simulink library "halout"  (R2021b)
settings: Solver=VariableStepAuto  StartTime=0.0  StopTime=10.0  RelTol=1e-3
undefined symbols (not defined in the file): C_TASK_5MS_S, FALSE, KHAL_CAN1FD1APS3E2E_flg, KHAL_CAN1FD1APS3TxReq_flg, KHAL_CAN1FD1VCU2E2E_flg, KHAL_CAN1FD1VCU2TxReq_flg, KHAL_CAN1FD1VCU3E2E_flg, KHAL_CAN1FD1VCU3TxReq_flg, KHAL_CAN1TxReq_flg, KHAL_CAN1VMCFCM1E2E_flg, KHAL_CAN1VMCFCM1TxReq_flg, KHAL_CAN2TxReq_flg, KHAL_CAN3FD3VCU1toNIDECTxReq_flg, KHAL_CAN3FD3VCU1TxReq_flg, KHAL_CAN3FD3VCU2E2E_flg, KHAL_CAN3FD3VCU2toNIDECE2E_flg, KHAL_CAN3FD3VCU2toNIDECTxReq_flg, KHAL_CAN3FD3VCU2TxReq_flg, KHAL_CAN3TxReq_flg, KHAL_CAN4FD4CE1000E2E_flg, KHAL_CAN4FD4CE1000TxReq_flg, KHAL_CAN4TxReq_flg, KHAL_CAN5TxReq_flg, KHAL_CAN6FD6APS3E2E_flg, KHAL_CAN6FD6APS3TxReq_flg, KHAL_CAN6FD6VCU2E2E_flg, KHAL_CAN6FD6VCU2TxReq_flg, KHAL_CAN6TxReq_flg, ONE_INT, TRUE, ZERO_INT
libraries: FVT_lib x549, simulink x244
(part 9 of 27)

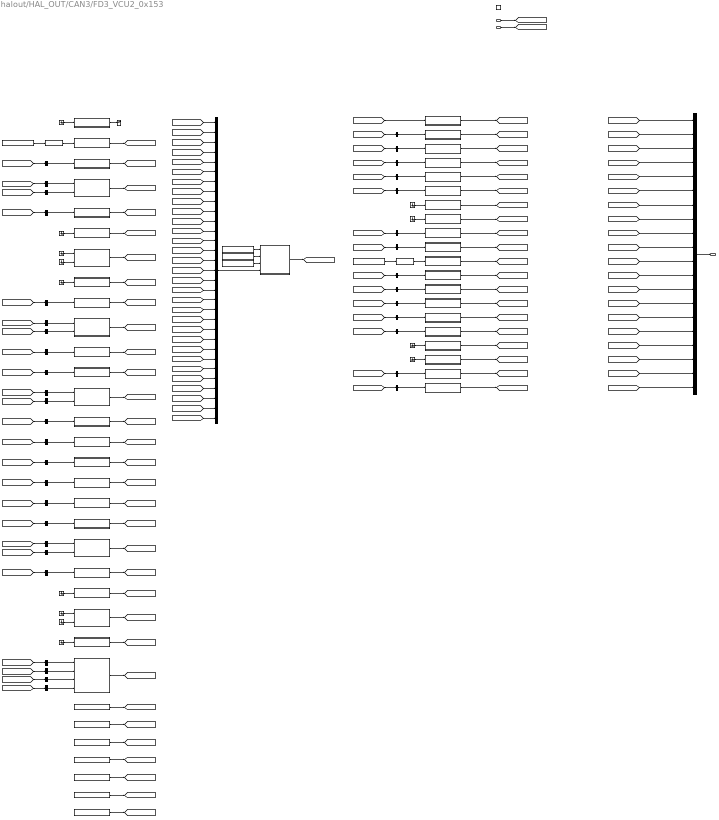
== system halout/HAL_OUT/CAN3/FD3_VCU2_0x153 ==
  BSCP_outputs : Inport  OutDataTypeStr=Bus: BSCP_outputs
  BOUTP_outputs : Inport  Port=2  OutDataTypeStr=Bus: BOUTP_outputs
  Trigger : TriggerPort  TriggerType=function-call  VariantControl=(inherit)
  Byte_0 : Subsystem
  Byte_1 : Subsystem
  Byte_10 : Subsystem
  Byte_11 : Subsystem
  Byte_12 : Subsystem
  Byte_13 : Subsystem
  Byte_14 : Subsystem
  Byte_15 : Subsystem
  Byte_16 : Subsystem
  Byte_17 : Subsystem
  Byte_18 : Subsystem
  Byte_19 : Subsystem
  Byte_2 : Subsystem
  Byte_20 : Subsystem
  Byte_21 : Subsystem
  Byte_22 : Subsystem
  Byte_23 : Subsystem
  Byte_24 : Subsystem
  Byte_{25..31} (7 alike) : Constant  Value=ZERO_INT
  Byte_3 : Subsystem
  Byte_4 : Subsystem
  Byte_5 : Subsystem
  Byte_6 : Subsystem
  Byte_7 : Subsystem
  Byte_8 : Subsystem
  Byte_9 : Subsystem
  CRC8_IfAction_Tx : Subsystem  AncestorBlock=FVT_lib/hal/CRC8_IfAction_Tx
      mask help: MeasumentTrigerEvent
      mask Display: fprintf('CRC8_IfAction');
  CSVCU2CAN1 : Subsystem
  Constant : Constant  Value=KHAL_CAN3FD3VCU2E2E_flg
  Constant1 : Constant  Value=0x40
  Constant2 : Constant  Value=0x24
  Constant3 : Constant  Value=KHAL_CAN3FD3VCU2E2E_flg
  Constant4 : Constant  Value=KHAL_CAN3FD3VCU2E2E_flg
  FrActvDmpDisabReq : Subsystem
  FrIdcMax : Subsystem
  FrIdcMin : Subsystem
  FrMCUEnaReq : Subsystem
  FrTMTqReq : Subsystem
  FrTorqMax : Subsystem
  FrTorqMin : Subsystem
  FrUdcMax : Subsystem
  FrUdcMin : Subsystem
  Ground{,1..12} (13 alike) : Ground
  Mux2 : Mux  Inputs=31
  RCVCU2CAN1 : Subsystem
  RollingCounter_IfAction : FVT_lib/hal/RollingCounter_IfAction
  RollingCounter_IfAction1 : FVT_lib/hal/RollingCounter_IfAction
  RrActvDmpDisabReq : Subsystem
  RrIdcMax : Subsystem
  RrIdcMin : Subsystem
  RrMCUEnaReq : Subsystem
  RrTMTqReq : Subsystem
  RrTorqMax : Subsystem
  RrTorqMin : Subsystem
  RrUdcMax : Subsystem
  RrUdcMin : Subsystem
  Terminator : Terminator
  bus_creator : BusCreator  Inputs=20  OutDataTypeStr=Bus: DT_CAN3_SG_FD3_VCU2  NonVirtualBus=on
  bus_selector : BusSelector  OutputSignals=VOUTP_RrIdcMax_A
  bus_selector1 : BusSelector  OutputSignals=VOUTP_RrIdcMax_A
  bus_selector10 : BusSelector  OutputSignals=VOUTP_FrUdcMin_V
  bus_selector11 : BusSelector  OutputSignals=VOUTP_FrUdcMin_V
  bus_selector12 : BusSelector  OutputSignals=VOUTP_RrTMTqReq_Nm
  bus_selector13 : BusSelector  OutputSignals=VOUTP_RrTMTqReq_Nm
  bus_selector14 : BusSelector  OutputSignals=VOUTP_FrTMTqReq_Nm
  bus_selector15 : BusSelector  OutputSignals=VOUTP_FrTMTqReq_Nm
  bus_selector16 : BusSelector  OutputSignals=VOUTP_FrIdcMax_A
  bus_selector17 : BusSelector  OutputSignals=VOUTP_FrIdcMax_A
  bus_selector18 : BusSelector  OutputSignals=VOUTP_FrIdcMin_A
  bus_selector19 : BusSelector  OutputSignals=VOUTP_FrIdcMin_A
  bus_selector2 : BusSelector  OutputSignals=VOUTP_RrIdcMin_A
  bus_selector20 : BusSelector  OutputSignals=VOUTP_FrActvDmpDisabReq_flg
  bus_selector21 : BusSelector  OutputSignals=VOUTP_FrMCUEnaReq_flg
  bus_selector22 : BusSelector  OutputSignals=VOUTP_RrActvDmpDisabReq_flg
  bus_selector23 : BusSelector  OutputSignals=VOUTP_RrMCUEnaReq_flg
  bus_selector24 : BusSelector  OutputSignals=VOUTP_FrActvDmpDisabReq_flg
  bus_selector25 : BusSelector  OutputSignals=VOUTP_FrIdcMax_A
  bus_selector26 : BusSelector  OutputSignals=VOUTP_FrIdcMin_A
  bus_selector27 : BusSelector  OutputSignals=VOUTP_FrMCUEnaReq_flg
  bus_selector28 : BusSelector  OutputSignals=VOUTP_FrTMTqReq_Nm
  bus_selector29 : BusSelector  OutputSignals=VOUTP_FrUdcMax_V
  bus_selector3 : BusSelector  OutputSignals=VOUTP_RrIdcMin_A
  bus_selector30 : BusSelector  OutputSignals=VOUTP_FrUdcMin_V
  bus_selector31 : BusSelector  OutputSignals=VOUTP_RrActvDmpDisabReq_flg
  bus_selector32 : BusSelector  OutputSignals=VOUTP_RrIdcMax_A
  bus_selector33 : BusSelector  OutputSignals=VOUTP_RrIdcMin_A
  bus_selector34 : BusSelector  OutputSignals=VOUTP_RrMCUEnaReq_flg
  bus_selector35 : BusSelector  OutputSignals=VOUTP_RrTMTqReq_Nm
  bus_selector36 : BusSelector  OutputSignals=VOUTP_RrUdcMax_V
  bus_selector37 : BusSelector  OutputSignals=VOUTP_RrUdcMin_V
  bus_selector4 : BusSelector  OutputSignals=VOUTP_RrUdcMax_V
  bus_selector5 : BusSelector  OutputSignals=VOUTP_RrUdcMax_V
  bus_selector6 : BusSelector  OutputSignals=VOUTP_RrUdcMin_V
  bus_selector7 : BusSelector  OutputSignals=VOUTP_RrUdcMin_V
  bus_selector8 : BusSelector  OutputSignals=VOUTP_FrUdcMax_V
  bus_selector9 : BusSelector  OutputSignals=VOUTP_FrUdcMax_V
  FD3_VCU2 : Outport
  wires:
  BSCP_outputs/1 -> [BSCP_outputs]
  BOUTP_outputs/1 -> [BOUTP_outputs]
  [CAN3_CS_VCU2_CAN1] -> bus_creator/1  "CAN3_CS_VCU2_CAN1"
  [CAN3_Fr_ActvDmpDisabReq] -> bus_creator/2  "CAN3_Fr_ActvDmpDisabReq"
  [CAN3_Fr_IdcMax] -> bus_creator/3  "CAN3_Fr_IdcMax"
  [CAN3_Fr_IdcMin] -> bus_creator/4  "CAN3_Fr_IdcMin"
  [CAN3_Fr_MCUEnaReq] -> bus_creator/5  "CAN3_Fr_MCUEnaReq"
  [CAN3_Fr_TMTqReq] -> bus_creator/6  "CAN3_Fr_TMTqReq"
  [CAN3_Fr_TorqMax] -> bus_creator/7  "CAN3_Fr_TorqMax"
  [CAN3_Fr_TorqMin] -> bus_creator/8  "CAN3_Fr_TorqMin"
  [CAN3_Fr_UdcMax] -> bus_creator/9  "CAN3_Fr_UdcMax"
  [CAN3_Fr_UdcMin] -> bus_creator/10  "CAN3_Fr_UdcMin"
  [CAN3_RC_VCU2_CAN1] -> bus_creator/11  "CAN3_RC_VCU2_CAN1"
  [CAN3_Rr_ActvDmpDisabReq] -> bus_creator/12  "CAN3_Rr_ActvDmpDisabReq"
  [CAN3_Rr_IdcMax] -> bus_creator/13  "CAN3_Rr_IdcMax"
  [CAN3_Rr_IdcMin] -> bus_creator/14  "CAN3_Rr_IdcMin"
  [CAN3_Rr_MCUEnaReq] -> bus_creator/15  "CAN3_Rr_MCUEnaReq"
  [CAN3_Rr_TMTqReq] -> bus_creator/16  "CAN3_Rr_TMTqReq"
  [CAN3_Rr_TorqMax] -> bus_creator/17  "CAN3_Rr_TorqMax"
  [CAN3_Rr_TorqMin] -> bus_creator/18  "CAN3_Rr_TorqMin"
  [CAN3_Rr_UdcMax] -> bus_creator/19  "CAN3_Rr_UdcMax"
  [CAN3_Rr_UdcMin] -> bus_creator/20  "CAN3_Rr_UdcMin"
  bus_creator/1 -> FD3_VCU2/1
  CSVCU2CAN1/1(CAN3_CS_VCU2_CAN1) -> [CAN3_CS_VCU2_CAN1]
  FrActvDmpDisabReq/1(CAN3_Fr_ActvDmpDisabReq) -> [CAN3_Fr_ActvDmpDisabReq]
  FrIdcMax/1(CAN3_Fr_IdcMax) -> [CAN3_Fr_IdcMax]
  FrIdcMin/1(CAN3_Fr_IdcMin) -> [CAN3_Fr_IdcMin]
  FrMCUEnaReq/1(CAN3_Fr_MCUEnaReq) -> [CAN3_Fr_MCUEnaReq]
  FrTMTqReq/1(CAN3_Fr_TMTqReq) -> [CAN3_Fr_TMTqReq]
  FrTorqMax/1(CAN3_Fr_TorqMax) -> [CAN3_Fr_TorqMax]
  FrTorqMin/1(CAN3_Fr_TorqMin) -> [CAN3_Fr_TorqMin]
  FrUdcMax/1(CAN3_Fr_UdcMax) -> [CAN3_Fr_UdcMax]
  FrUdcMin/1(CAN3_Fr_UdcMin) -> [CAN3_Fr_UdcMin]
  RCVCU2CAN1/1(CAN3_RC_VCU2_CAN1) -> [CAN3_RC_VCU2_CAN1]
  RrActvDmpDisabReq/1(CAN3_Rr_ActvDmpDisabReq) -> [CAN3_Rr_ActvDmpDisabReq]
  RrIdcMax/1(CAN3_Rr_IdcMax) -> [CAN3_Rr_IdcMax]
  RrIdcMin/1(CAN3_Rr_IdcMin) -> [CAN3_Rr_IdcMin]
  RrMCUEnaReq/1(CAN3_Rr_MCUEnaReq) -> [CAN3_Rr_MCUEnaReq]
  RrTMTqReq/1(CAN3_Rr_TMTqReq) -> [CAN3_Rr_TMTqReq]
  RrTorqMax/1(CAN3_Rr_TorqMax) -> [CAN3_Rr_TorqMax]
  RrTorqMin/1(CAN3_Rr_TorqMin) -> [CAN3_Rr_TorqMin]
  RrUdcMax/1(CAN3_Rr_UdcMax) -> [CAN3_Rr_UdcMax]
  RrUdcMin/1(CAN3_Rr_UdcMin) -> [CAN3_Rr_UdcMin]
  Byte_0/1(Byte_0) -> Terminator/1
  Byte_1/1(Byte_1) -> [Byte_1]
  Byte_2/1(Byte_2) -> [Byte_2]
  Byte_3/1(Byte_3) -> [Byte_3]
  Byte_4/1(Byte_4) -> [Byte_4]
  Byte_5/1(Byte_5) -> [Byte_5]
  Byte_6/1(Byte_6) -> [Byte_6]
  Byte_7/1(Byte_7) -> [Byte_7]
  Byte_8/1(Byte_8) -> [Byte_8]
  Byte_9/1(Byte_9) -> [Byte_9]
  Byte_10/1(Byte_10) -> [Byte_10]
  Byte_11/1(Byte_11) -> [Byte_11]
  Byte_12/1(Byte_12) -> [Byte_12]
  Byte_13/1(Byte_13) -> [Byte_13]
  Byte_14/1(Byte_14) -> [Byte_14]
  Byte_15/1(Byte_15) -> [Byte_15]
  Byte_16/1(Byte_16) -> [Byte_16]
  Byte_17/1(Byte_17) -> [Byte_17]
  Byte_18/1(Byte_18) -> [Byte_18]
  Byte_19/1(Byte_19) -> [Byte_19]
  Byte_20/1(Byte_20) -> [Byte_20]
  Byte_21/1(Byte_21) -> [Byte_21]
  Byte_22/1(Byte_22) -> [Byte_22]
  Byte_23/1(Byte_23) -> [Byte_23]
  Byte_24/1(Byte_24) -> [Byte_24]
  Byte_25/1 -> [Byte_25]
  Byte_26/1 -> [Byte_26]
  Byte_27/1 -> [Byte_27]
  Byte_28/1 -> [Byte_28]
  Byte_29/1 -> [Byte_29]
  Byte_30/1 -> [Byte_30]
  Byte_31/1 -> [Byte_31]
  Mux2/1 -> CRC8_IfAction_Tx/4(RawData)
  Constant/1 -> CRC8_IfAction_Tx/1(CAN_E2E_flg)
  Constant1/1 -> CRC8_IfAction_Tx/2(DataID1)
  Constant2/1 -> CRC8_IfAction_Tx/3(DataID2)
  CRC8_IfAction_Tx/1(CRC8) -> [CS_VCU2_CAN1]
  Ground/1 -> Byte_0/1(CS_VCU2_CAN1)
  [Byte_1] -> Mux2/1
  RollingCounter_IfAction/1 -> Byte_1/1(RC_VCU2_CAN1)
  Constant3/1 -> RollingCounter_IfAction/1
  [Byte_2] -> Mux2/2
  bus_selector/1 -> Byte_2/1(Rr_IdcMax)  "<VOUTP_RrIdcMax_A>"
  [BOUTP_outputs] -> bus_selector/1
  [Byte_3] -> Mux2/3
  bus_selector1/1 -> Byte_3/1(Rr_IdcMax)  "<VOUTP_RrIdcMax_A>"
  [BOUTP_outputs] -> bus_selector1/1
  bus_selector2/1 -> Byte_3/2(Rr_IdcMin)  "<VOUTP_RrIdcMin_A>"
  [BOUTP_outputs] -> bus_selector2/1
  [Byte_4] -> Mux2/4
  bus_selector3/1 -> Byte_4/1(Rr_IdcMin)  "<VOUTP_RrIdcMin_A>"
  [BOUTP_outputs] -> bus_selector3/1
  [Byte_5] -> Mux2/5
  Ground1/1 -> Byte_5/1(Rr_TorqMax)
  [Byte_6] -> Mux2/6
  Ground2/1 -> Byte_6/1(Rr_TorqMax)
  Ground3/1 -> Byte_6/2(Rr_TorqMin)
  [Byte_7] -> Mux2/7
  Ground4/1 -> Byte_7/1(Rr_TorqMin)
  [Byte_8] -> Mux2/8
  bus_selector4/1 -> Byte_8/1(Rr_UdcMax)  "<VOUTP_RrUdcMax_V>"
  [BOUTP_outputs] -> bus_selector4/1
  [Byte_9] -> Mux2/9
  bus_selector5/1 -> Byte_9/1(Rr_UdcMax)  "<VOUTP_RrUdcMax_V>"
  [BOUTP_outputs] -> bus_selector5/1
  bus_selector6/1 -> Byte_9/2(Rr_UdcMin)  "<VOUTP_RrUdcMin_V>"
  [BOUTP_outputs] -> bus_selector6/1
  [Byte_10] -> Mux2/10
  bus_selector7/1 -> Byte_10/1(Rr_UdcMin)  "<VOUTP_RrUdcMin_V>"
  [BOUTP_outputs] -> bus_selector7/1
  [Byte_11] -> Mux2/11
  bus_selector8/1 -> Byte_11/1(Fr_UdcMax)  "<VOUTP_FrUdcMax_V>"
  [BOUTP_outputs] -> bus_selector8/1
  [Byte_12] -> Mux2/12
  bus_selector9/1 -> Byte_12/1(Fr_UdcMax)  "<VOUTP_FrUdcMax_V>"
  [BOUTP_outputs] -> bus_selector9/1
  bus_selector10/1 -> Byte_12/2(Fr_UdcMin)  "<VOUTP_FrUdcMin_V>"
  [BOUTP_outputs] -> bus_selector10/1
  [Byte_13] -> Mux2/13
  bus_selector11/1 -> Byte_13/1(Fr_UdcMin)  "<VOUTP_FrUdcMin_V>"
  [BOUTP_outputs] -> bus_selector11/1
  [Byte_14] -> Mux2/14
  bus_selector12/1 -> Byte_14/1(Rr_TMTqReq)  "<VOUTP_RrTMTqReq_Nm>"
  [BOUTP_outputs] -> bus_selector12/1
  [Byte_15] -> Mux2/15
  bus_selector13/1 -> Byte_15/1(Rr_TMTqReq)  "<VOUTP_RrTMTqReq_Nm>"
  [BOUTP_outputs] -> bus_selector13/1
  [Byte_16] -> Mux2/16
  bus_selector14/1 -> Byte_16/1(Fr_TMTqReq)  "<VOUTP_FrTMTqReq_Nm>"
  [BOUTP_outputs] -> bus_selector14/1
  [Byte_17] -> Mux2/17
  bus_selector15/1 -> Byte_17/1(Fr_TMTqReq)  "<VOUTP_FrTMTqReq_Nm>"
  [BOUTP_outputs] -> bus_selector15/1
  [Byte_18] -> Mux2/18
  bus_selector16/1 -> Byte_18/1(Fr_IdcMax)  "<VOUTP_FrIdcMax_A>"
  [BOUTP_outputs] -> bus_selector16/1
  [Byte_19] -> Mux2/19
  bus_selector17/1 -> Byte_19/1(Fr_IdcMax)  "<VOUTP_FrIdcMax_A>"
  [BOUTP_outputs] -> bus_selector17/1
  bus_selector18/1 -> Byte_19/2(Fr_IdcMin)  "<VOUTP_FrIdcMin_A>"
  [BOUTP_outputs] -> bus_selector18/1
  [Byte_20] -> Mux2/20
  bus_selector19/1 -> Byte_20/1(Fr_IdcMin)  "<VOUTP_FrIdcMin_A>"
  [BOUTP_outputs] -> bus_selector19/1
  [Byte_21] -> Mux2/21
  Ground5/1 -> Byte_21/1(Fr_TorqMax)
  [Byte_22] -> Mux2/22
  Ground6/1 -> Byte_22/1(Fr_TorqMax)
  Ground7/1 -> Byte_22/2(Fr_TorqMin)
  [Byte_23] -> Mux2/23
  Ground8/1 -> Byte_23/1(Fr_TorqMin)
  [Byte_24] -> Mux2/24
  bus_selector20/1 -> Byte_24/1(Fr_ActvDmpDisabReq)  "<VOUTP_FrActvDmpDisabReq_flg>"
  [BOUTP_outputs] -> bus_selector20/1
  bus_selector21/1 -> Byte_24/2(Fr_MCUEnaReq)  "<VOUTP_FrMCUEnaReq_flg>"
  [BOUTP_outputs] -> bus_selector21/1
  bus_selector22/1 -> Byte_24/3(Rr_ActvDmpDisabReq)  "<VOUTP_RrActvDmpDisabReq_flg>"
  [BOUTP_outputs] -> bus_selector22/1
  bus_selector23/1 -> Byte_24/4(Rr_MCUEnaReq)  "<VOUTP_RrMCUEnaReq_flg>"
  [BOUTP_outputs] -> bus_selector23/1
  [Byte_25] -> Mux2/25
  [Byte_26] -> Mux2/26
  [Byte_27] -> Mux2/27
  [Byte_28] -> Mux2/28
  [Byte_29] -> Mux2/29
  [Byte_30] -> Mux2/30
  [Byte_31] -> Mux2/31
  [CS_VCU2_CAN1] -> CSVCU2CAN1/1(CSVCU2CAN1)
  bus_selector24/1 -> FrActvDmpDisabReq/1(FrActvDmpDisabReq)  "<VOUTP_FrActvDmpDisabReq_flg>"
  [BOUTP_outputs] -> bus_selector24/1
  bus_selector25/1 -> FrIdcMax/1(FrIdcMax)  "<VOUTP_FrIdcMax_A>"
  [BOUTP_outputs] -> bus_selector25/1
  bus_selector26/1 -> FrIdcMin/1(FrIdcMin)  "<VOUTP_FrIdcMin_A>"
  [BOUTP_outputs] -> bus_selector26/1
  bus_selector27/1 -> FrMCUEnaReq/1(FrMCUEnaReq)  "<VOUTP_FrMCUEnaReq_flg>"
  [BOUTP_outputs] -> bus_selector27/1
  bus_selector28/1 -> FrTMTqReq/1(FrTMTqReq)  "<VOUTP_FrTMTqReq_Nm>"
  [BOUTP_outputs] -> bus_selector28/1
  Ground9/1 -> FrTorqMax/1(FrTorqMax)
  Ground10/1 -> FrTorqMin/1(FrTorqMin)
  bus_selector29/1 -> FrUdcMax/1(FrUdcMax)  "<VOUTP_FrUdcMax_V>"
  [BOUTP_outputs] -> bus_selector29/1
  bus_selector30/1 -> FrUdcMin/1(FrUdcMin)  "<VOUTP_FrUdcMin_V>"
  [BOUTP_outputs] -> bus_selector30/1
  RollingCounter_IfAction1/1 -> RCVCU2CAN1/1(RCVCU2CAN1)
  Constant4/1 -> RollingCounter_IfAction1/1
  bus_selector31/1 -> RrActvDmpDisabReq/1(RrActvDmpDisabReq)  "<VOUTP_RrActvDmpDisabReq_flg>"
  [BOUTP_outputs] -> bus_selector31/1
  bus_selector32/1 -> RrIdcMax/1(RrIdcMax)  "<VOUTP_RrIdcMax_A>"
  [BOUTP_outputs] -> bus_selector32/1
  bus_selector33/1 -> RrIdcMin/1(RrIdcMin)  "<VOUTP_RrIdcMin_A>"
  [BOUTP_outputs] -> bus_selector33/1
  bus_selector34/1 -> RrMCUEnaReq/1(RrMCUEnaReq)  "<VOUTP_RrMCUEnaReq_flg>"
  [BOUTP_outputs] -> bus_selector34/1
  bus_selector35/1 -> RrTMTqReq/1(RrTMTqReq)  "<VOUTP_RrTMTqReq_Nm>"
  [BOUTP_outputs] -> bus_selector35/1
  Ground11/1 -> RrTorqMax/1(RrTorqMax)
  Ground12/1 -> RrTorqMin/1(RrTorqMin)
  bus_selector36/1 -> RrUdcMax/1(RrUdcMax)  "<VOUTP_RrUdcMax_V>"
  [BOUTP_outputs] -> bus_selector36/1
  bus_selector37/1 -> RrUdcMin/1(RrUdcMin)  "<VOUTP_RrUdcMin_V>"
  [BOUTP_outputs] -> bus_selector37/1

== system halout/HAL_OUT/CAN3/FD3_VCU2_Tx ==
  TxReq : Inport
  Chart : Stateflow chart  TreatAsAtomicUnit=on
  Constant : Constant  Value=C_TASK_5MS_S
  Constant3 : Constant  Value=CycleTime
  Data Type Conversion : DataTypeConversion  OutDataTypeStr=uint16
  Divide : Product  Inputs=*/
  Gain : Gain  Gain=0.001
  TxTrigger : Outport
  wires:
  Data Type Conversion/1 -> Chart/2(CycleCnt)
  Constant3/1 -> Gain/1
  Gain/1 -> Divide/1
  Chart/1(TxTrigger()) -> TxTrigger/1
  Divide/1 -> Data Type Conversion/1
  TxReq/1 -> Chart/1(TxReq)
  Constant/1 -> Divide/2

== system halout/HAL_OUT/CAN3/FD3_VCU2_toNIDEC_0x154 ==
  BSCP_outputs : Inport  OutDataTypeStr=Bus: BSCP_outputs
  BOUTP_outputs : Inport  Port=2  OutDataTypeStr=Bus: BOUTP_outputs
  Trigger : TriggerPort  TriggerType=function-call  VariantControl=(inherit)
  Byte_0 : Subsystem
  Byte_1 : Subsystem
  Byte_10 : Subsystem
  Byte_11 : Subsystem
  Byte_12 : Subsystem
  Byte_13 : Subsystem
  Byte_14 : Subsystem
  Byte_15 : Subsystem
  Byte_16 : Subsystem
  Byte_17 : Subsystem
  Byte_18 : Subsystem
  Byte_19 : Subsystem
  Byte_2 : Subsystem
  Byte_20 : Subsystem
  Byte_21 : Subsystem
  Byte_22 : Subsystem
  Byte_23 : Subsystem
  Byte_3 : Subsystem
  Byte_4 : Subsystem
  Byte_5 : Subsystem
  Byte_6 : Subsystem
  Byte_7 : Subsystem
  Byte_8 : Subsystem
  Byte_9 : Subsystem
  CRC8_IfAction_Tx : Subsystem  AncestorBlock=FVT_lib/hal/CRC8_IfAction_Tx
      mask help: MeasumentTrigerEvent
      mask Display: fprintf('CRC8_IfAction');
  CSVCU2CAN1toNidec : Subsystem
  Constant : Constant  Value=KHAL_CAN3FD3VCU2toNIDECE2E_flg
  Constant1 : Constant  Value=0x41
  Constant2 : Constant  Value=0x14
  Constant3 : Constant  Value=KHAL_CAN3FD3VCU2toNIDECE2E_flg
  Constant4 : Constant  Value=KHAL_CAN3FD3VCU2toNIDECE2E_flg
  FrIdcMaxtoNidec : Subsystem
  FrIdcMintoNidec : Subsystem
  FrTMTqReqtoNidec : Subsystem
  FrTorqMaxtoNidec : Subsystem
  FrTorqMintoNidec : Subsystem
  FrUdcMaxtoNidec : Subsystem
  FrUdcMintoNidec : Subsystem
  Ground{,1..12} (13 alike) : Ground
  Mux2 : Mux  Inputs=23
  RCVCU2CAN1toNidec : Subsystem
  RollingCounter_IfAction : FVT_lib/hal/RollingCounter_IfAction
  RollingCounter_IfAction1 : FVT_lib/hal/RollingCounter_IfAction
  RrIdcMaxtoNidec : Subsystem
  RrIdcMintoNidec : Subsystem
  RrTMTqReqtoNidec : Subsystem
  RrTorqMaxtoNidec : Subsystem
  RrTorqMintoNidec : Subsystem
  RrUdcMaxtoNidec : Subsystem
  RrUdcMintoNidec : Subsystem
  Terminator : Terminator
  bus_creator : BusCreator  Inputs=16  OutDataTypeStr=Bus: DT_CAN3_SG_FD3_VCU2_toNIDEC  NonVirtualBus=on
  bus_selector : BusSelector  OutputSignals=VOUTP_RrIdcMax_A
  bus_selector1 : BusSelector  OutputSignals=VOUTP_RrIdcMax_A
  bus_selector10 : BusSelector  OutputSignals=VOUTP_FrUdcMin_V
  bus_selector11 : BusSelector  OutputSignals=VOUTP_FrUdcMin_V
  bus_selector12 : BusSelector  OutputSignals=VOUTP_RrTMTqReq_Nm
  bus_selector13 : BusSelector  OutputSignals=VOUTP_RrTMTqReq_Nm
  bus_selector14 : BusSelector  OutputSignals=VOUTP_FrTMTqReq_Nm
  bus_selector15 : BusSelector  OutputSignals=VOUTP_FrTMTqReq_Nm
  bus_selector16 : BusSelector  OutputSignals=VOUTP_FrIdcMax_A
  bus_selector17 : BusSelector  OutputSignals=VOUTP_FrIdcMax_A
  bus_selector18 : BusSelector  OutputSignals=VOUTP_FrIdcMin_A
  bus_selector19 : BusSelector  OutputSignals=VOUTP_FrIdcMin_A
  bus_selector2 : BusSelector  OutputSignals=VOUTP_RrIdcMin_A
  bus_selector20 : BusSelector  OutputSignals=VOUTP_FrIdcMax_A
  bus_selector21 : BusSelector  OutputSignals=VOUTP_FrIdcMin_A
  bus_selector22 : BusSelector  OutputSignals=VOUTP_FrTMTqReq_Nm
  bus_selector23 : BusSelector  OutputSignals=VOUTP_FrUdcMax_V
  bus_selector24 : BusSelector  OutputSignals=VOUTP_FrUdcMin_V
  bus_selector25 : BusSelector  OutputSignals=VOUTP_RrIdcMax_A
  bus_selector26 : BusSelector  OutputSignals=VOUTP_RrIdcMin_A
  bus_selector27 : BusSelector  OutputSignals=VOUTP_RrTMTqReq_Nm
  bus_selector28 : BusSelector  OutputSignals=VOUTP_RrUdcMax_V
  bus_selector29 : BusSelector  OutputSignals=VOUTP_RrUdcMin_V
  bus_selector3 : BusSelector  OutputSignals=VOUTP_RrIdcMin_A
  bus_selector4 : BusSelector  OutputSignals=VOUTP_RrUdcMax_V
  bus_selector5 : BusSelector  OutputSignals=VOUTP_RrUdcMax_V
  bus_selector6 : BusSelector  OutputSignals=VOUTP_RrUdcMin_V
  bus_selector7 : BusSelector  OutputSignals=VOUTP_RrUdcMin_V
  bus_selector8 : BusSelector  OutputSignals=VOUTP_FrUdcMax_V
  bus_selector9 : BusSelector  OutputSignals=VOUTP_FrUdcMax_V
  FD3_VCU2_toNIDEC : Outport
  wires:
  BSCP_outputs/1 -> [BSCP_outputs]
  BOUTP_outputs/1 -> [BOUTP_outputs]
  [CAN3_CS_VCU2_CAN1_toNidec] -> bus_creator/1  "CAN3_CS_VCU2_CAN1_toNidec"
  [CAN3_Fr_IdcMax_toNidec] -> bus_creator/2  "CAN3_Fr_IdcMax_toNidec"
  [CAN3_Fr_IdcMin_toNidec] -> bus_creator/3  "CAN3_Fr_IdcMin_toNidec"
  [CAN3_Fr_TMTqReq_toNidec] -> bus_creator/4  "CAN3_Fr_TMTqReq_toNidec"
  [CAN3_Fr_TorqMax_toNidec] -> bus_creator/5  "CAN3_Fr_TorqMax_toNidec"
  [CAN3_Fr_TorqMin_toNidec] -> bus_creator/6  "CAN3_Fr_TorqMin_toNidec"
  [CAN3_Fr_UdcMax_toNidec] -> bus_creator/7  "CAN3_Fr_UdcMax_toNidec"
  [CAN3_Fr_UdcMin_toNidec] -> bus_creator/8  "CAN3_Fr_UdcMin_toNidec"
  [CAN3_RC_VCU2_CAN1_toNidec] -> bus_creator/9  "CAN3_RC_VCU2_CAN1_toNidec"
  [CAN3_Rr_IdcMax_toNidec] -> bus_creator/10  "CAN3_Rr_IdcMax_toNidec"
  [CAN3_Rr_IdcMin_toNidec] -> bus_creator/11  "CAN3_Rr_IdcMin_toNidec"
  [CAN3_Rr_TMTqReq_toNidec] -> bus_creator/12  "CAN3_Rr_TMTqReq_toNidec"
  [CAN3_Rr_TorqMax_toNidec] -> bus_creator/13  "CAN3_Rr_TorqMax_toNidec"
  [CAN3_Rr_TorqMin_toNidec] -> bus_creator/14  "CAN3_Rr_TorqMin_toNidec"
  [CAN3_Rr_UdcMax_toNidec] -> bus_creator/15  "CAN3_Rr_UdcMax_toNidec"
  [CAN3_Rr_UdcMin_toNidec] -> bus_creator/16  "CAN3_Rr_UdcMin_toNidec"
  bus_creator/1 -> FD3_VCU2_toNIDEC/1
  CSVCU2CAN1toNidec/1(CAN3_CS_VCU2_CAN1_toNidec) -> [CAN3_CS_VCU2_CAN1_toNidec]
  FrIdcMaxtoNidec/1(CAN3_Fr_IdcMax_toNidec) -> [CAN3_Fr_IdcMax_toNidec]
  FrIdcMintoNidec/1(CAN3_Fr_IdcMin_toNidec) -> [CAN3_Fr_IdcMin_toNidec]
  FrTMTqReqtoNidec/1(CAN3_Fr_TMTqReq_toNidec) -> [CAN3_Fr_TMTqReq_toNidec]
  FrTorqMaxtoNidec/1(CAN3_Fr_TorqMax_toNidec) -> [CAN3_Fr_TorqMax_toNidec]
  FrTorqMintoNidec/1(CAN3_Fr_TorqMin_toNidec) -> [CAN3_Fr_TorqMin_toNidec]
  FrUdcMaxtoNidec/1(CAN3_Fr_UdcMax_toNidec) -> [CAN3_Fr_UdcMax_toNidec]
  FrUdcMintoNidec/1(CAN3_Fr_UdcMin_toNidec) -> [CAN3_Fr_UdcMin_toNidec]
  RCVCU2CAN1toNidec/1(CAN3_RC_VCU2_CAN1_toNidec) -> [CAN3_RC_VCU2_CAN1_toNidec]
  RrIdcMaxtoNidec/1(CAN3_Rr_IdcMax_toNidec) -> [CAN3_Rr_IdcMax_toNidec]
  RrIdcMintoNidec/1(CAN3_Rr_IdcMin_toNidec) -> [CAN3_Rr_IdcMin_toNidec]
  RrTMTqReqtoNidec/1(CAN3_Rr_TMTqReq_toNidec) -> [CAN3_Rr_TMTqReq_toNidec]
  RrTorqMaxtoNidec/1(CAN3_Rr_TorqMax_toNidec) -> [CAN3_Rr_TorqMax_toNidec]
  RrTorqMintoNidec/1(CAN3_Rr_TorqMin_toNidec) -> [CAN3_Rr_TorqMin_toNidec]
  RrUdcMaxtoNidec/1(CAN3_Rr_UdcMax_toNidec) -> [CAN3_Rr_UdcMax_toNidec]
  RrUdcMintoNidec/1(CAN3_Rr_UdcMin_toNidec) -> [CAN3_Rr_UdcMin_toNidec]
  Byte_0/1(Byte_0) -> Terminator/1
  Byte_1/1(Byte_1) -> [Byte_1]
  Byte_2/1(Byte_2) -> [Byte_2]
  Byte_3/1(Byte_3) -> [Byte_3]
  Byte_4/1(Byte_4) -> [Byte_4]
  Byte_5/1(Byte_5) -> [Byte_5]
  Byte_6/1(Byte_6) -> [Byte_6]
  Byte_7/1(Byte_7) -> [Byte_7]
  Byte_8/1(Byte_8) -> [Byte_8]
  Byte_9/1(Byte_9) -> [Byte_9]
  Byte_10/1(Byte_10) -> [Byte_10]
  Byte_11/1(Byte_11) -> [Byte_11]
  Byte_12/1(Byte_12) -> [Byte_12]
  Byte_13/1(Byte_13) -> [Byte_13]
  Byte_14/1(Byte_14) -> [Byte_14]
  Byte_15/1(Byte_15) -> [Byte_15]
  Byte_16/1(Byte_16) -> [Byte_16]
  Byte_17/1(Byte_17) -> [Byte_17]
  Byte_18/1(Byte_18) -> [Byte_18]
  Byte_19/1(Byte_19) -> [Byte_19]
  Byte_20/1(Byte_20) -> [Byte_20]
  Byte_21/1(Byte_21) -> [Byte_21]
  Byte_22/1(Byte_22) -> [Byte_22]
  Byte_23/1(Byte_23) -> [Byte_23]
  Mux2/1 -> CRC8_IfAction_Tx/4(RawData)
  Constant/1 -> CRC8_IfAction_Tx/1(CAN_E2E_flg)
  Constant1/1 -> CRC8_IfAction_Tx/2(DataID1)
  Constant2/1 -> CRC8_IfAction_Tx/3(DataID2)
  CRC8_IfAction_Tx/1(CRC8) -> [CS_VCU2_CAN1_toNidec]
  Ground/1 -> Byte_0/1(CS_VCU2_CAN1_toNidec)
  [Byte_1] -> Mux2/1
  RollingCounter_IfAction/1 -> Byte_1/1(RC_VCU2_CAN1_toNidec)
  Constant3/1 -> RollingCounter_IfAction/1
  [Byte_2] -> Mux2/2
  bus_selector/1 -> Byte_2/1(Rr_IdcMax_toNidec)  "<VOUTP_RrIdcMax_A>"
  [BOUTP_outputs] -> bus_selector/1
  [Byte_3] -> Mux2/3
  bus_selector1/1 -> Byte_3/1(Rr_IdcMax_toNidec)  "<VOUTP_RrIdcMax_A>"
  [BOUTP_outputs] -> bus_selector1/1
  bus_selector2/1 -> Byte_3/2(Rr_IdcMin_toNidec)  "<VOUTP_RrIdcMin_A>"
  [BOUTP_outputs] -> bus_selector2/1
  [Byte_4] -> Mux2/4
  bus_selector3/1 -> Byte_4/1(Rr_IdcMin_toNidec)  "<VOUTP_RrIdcMin_A>"
  [BOUTP_outputs] -> bus_selector3/1
  [Byte_5] -> Mux2/5
  Ground1/1 -> Byte_5/1(Rr_TorqMax_toNidec)
  [Byte_6] -> Mux2/6
  Ground2/1 -> Byte_6/1(Rr_TorqMax_toNidec)
  Ground3/1 -> Byte_6/2(Rr_TorqMin_toNidec)
  [Byte_7] -> Mux2/7
  Ground4/1 -> Byte_7/1(Rr_TorqMin_toNidec)
  [Byte_8] -> Mux2/8
  bus_selector4/1 -> Byte_8/1(Rr_UdcMax_toNidec)  "<VOUTP_RrUdcMax_V>"
  [BOUTP_outputs] -> bus_selector4/1
  [Byte_9] -> Mux2/9
  bus_selector5/1 -> Byte_9/1(Rr_UdcMax_toNidec)  "<VOUTP_RrUdcMax_V>"
  [BOUTP_outputs] -> bus_selector5/1
  bus_selector6/1 -> Byte_9/2(Rr_UdcMin_toNidec)  "<VOUTP_RrUdcMin_V>"
  [BOUTP_outputs] -> bus_selector6/1
  [Byte_10] -> Mux2/10
  bus_selector7/1 -> Byte_10/1(Rr_UdcMin_toNidec)  "<VOUTP_RrUdcMin_V>"
  [BOUTP_outputs] -> bus_selector7/1
  [Byte_11] -> Mux2/11
  bus_selector8/1 -> Byte_11/1(Fr_UdcMax_toNidec)  "<VOUTP_FrUdcMax_V>"
  [BOUTP_outputs] -> bus_selector8/1
  [Byte_12] -> Mux2/12
  bus_selector9/1 -> Byte_12/1(Fr_UdcMax_toNidec)  "<VOUTP_FrUdcMax_V>"
  [BOUTP_outputs] -> bus_selector9/1
  bus_selector10/1 -> Byte_12/2(Fr_UdcMin_toNidec)  "<VOUTP_FrUdcMin_V>"
  [BOUTP_outputs] -> bus_selector10/1
  [Byte_13] -> Mux2/13
  bus_selector11/1 -> Byte_13/1(Fr_UdcMin_toNidec)  "<VOUTP_FrUdcMin_V>"
  [BOUTP_outputs] -> bus_selector11/1
  [Byte_14] -> Mux2/14
  bus_selector12/1 -> Byte_14/1(Rr_TMTqReq_toNidec)  "<VOUTP_RrTMTqReq_Nm>"
  [BOUTP_outputs] -> bus_selector12/1
  [Byte_15] -> Mux2/15
  bus_selector13/1 -> Byte_15/1(Rr_TMTqReq_toNidec)  "<VOUTP_RrTMTqReq_Nm>"
  [BOUTP_outputs] -> bus_selector13/1
  [Byte_16] -> Mux2/16
  bus_selector14/1 -> Byte_16/1(Fr_TMTqReq_toNidec)  "<VOUTP_FrTMTqReq_Nm>"
  [BOUTP_outputs] -> bus_selector14/1
  [Byte_17] -> Mux2/17
  bus_selector15/1 -> Byte_17/1(Fr_TMTqReq_toNidec)  "<VOUTP_FrTMTqReq_Nm>"
  [BOUTP_outputs] -> bus_selector15/1
  [Byte_18] -> Mux2/18
  bus_selector16/1 -> Byte_18/1(Fr_IdcMax_toNidec)  "<VOUTP_FrIdcMax_A>"
  [BOUTP_outputs] -> bus_selector16/1
  [Byte_19] -> Mux2/19
  bus_selector17/1 -> Byte_19/1(Fr_IdcMax_toNidec)  "<VOUTP_FrIdcMax_A>"
  [BOUTP_outputs] -> bus_selector17/1
  bus_selector18/1 -> Byte_19/2(Fr_IdcMin_toNidec)  "<VOUTP_FrIdcMin_A>"
  [BOUTP_outputs] -> bus_selector18/1
  [Byte_20] -> Mux2/20
  bus_selector19/1 -> Byte_20/1(Fr_IdcMin_toNidec)  "<VOUTP_FrIdcMin_A>"
  [BOUTP_outputs] -> bus_selector19/1
  [Byte_21] -> Mux2/21
  Ground5/1 -> Byte_21/1(Fr_TorqMax_toNidec)
  [Byte_22] -> Mux2/22
  Ground6/1 -> Byte_22/1(Fr_TorqMax_toNidec)
  Ground7/1 -> Byte_22/2(Fr_TorqMin_toNidec)
  [Byte_23] -> Mux2/23
  Ground8/1 -> Byte_23/1(Fr_TorqMin_toNidec)
  [CS_VCU2_CAN1_toNidec] -> CSVCU2CAN1toNidec/1(CSVCU2CAN1toNidec)
  bus_selector20/1 -> FrIdcMaxtoNidec/1(FrIdcMaxtoNidec)  "<VOUTP_FrIdcMax_A>"
  [BOUTP_outputs] -> bus_selector20/1
  bus_selector21/1 -> FrIdcMintoNidec/1(FrIdcMintoNidec)  "<VOUTP_FrIdcMin_A>"
  [BOUTP_outputs] -> bus_selector21/1
  bus_selector22/1 -> FrTMTqReqtoNidec/1(FrTMTqReqtoNidec)  "<VOUTP_FrTMTqReq_Nm>"
  [BOUTP_outputs] -> bus_selector22/1
  Ground9/1 -> FrTorqMaxtoNidec/1(FrTorqMaxtoNidec)
  Ground10/1 -> FrTorqMintoNidec/1(FrTorqMintoNidec)
  bus_selector23/1 -> FrUdcMaxtoNidec/1(FrUdcMaxtoNidec)  "<VOUTP_FrUdcMax_V>"
  [BOUTP_outputs] -> bus_selector23/1
  bus_selector24/1 -> FrUdcMintoNidec/1(FrUdcMintoNidec)  "<VOUTP_FrUdcMin_V>"
  [BOUTP_outputs] -> bus_selector24/1
  RollingCounter_IfAction1/1 -> RCVCU2CAN1toNidec/1(RCVCU2CAN1toNidec)
  Constant4/1 -> RollingCounter_IfAction1/1
  bus_selector25/1 -> RrIdcMaxtoNidec/1(RrIdcMaxtoNidec)  "<VOUTP_RrIdcMax_A>"
  [BOUTP_outputs] -> bus_selector25/1
  bus_selector26/1 -> RrIdcMintoNidec/1(RrIdcMintoNidec)  "<VOUTP_RrIdcMin_A>"
  [BOUTP_outputs] -> bus_selector26/1
  bus_selector27/1 -> RrTMTqReqtoNidec/1(RrTMTqReqtoNidec)  "<VOUTP_RrTMTqReq_Nm>"
  [BOUTP_outputs] -> bus_selector27/1
  Ground11/1 -> RrTorqMaxtoNidec/1(RrTorqMaxtoNidec)
  Ground12/1 -> RrTorqMintoNidec/1(RrTorqMintoNidec)
  bus_selector28/1 -> RrUdcMaxtoNidec/1(RrUdcMaxtoNidec)  "<VOUTP_RrUdcMax_V>"
  [BOUTP_outputs] -> bus_selector28/1
  bus_selector29/1 -> RrUdcMintoNidec/1(RrUdcMintoNidec)  "<VOUTP_RrUdcMin_V>"
  [BOUTP_outputs] -> bus_selector29/1

== system halout/HAL_OUT/CAN3/FD3_VCU2_toNIDEC_Tx ==
  TxReq : Inport
  Chart : Stateflow chart  TreatAsAtomicUnit=on
  Constant : Constant  Value=C_TASK_5MS_S
  Constant3 : Constant  Value=CycleTime
  Data Type Conversion : DataTypeConversion  OutDataTypeStr=uint16
  Divide : Product  Inputs=*/
  Gain : Gain  Gain=0.001
  TxTrigger : Outport
  wires:
  Data Type Conversion/1 -> Chart/2(CycleCnt)
  Constant3/1 -> Gain/1
  Gain/1 -> Divide/1
  Chart/1(TxTrigger()) -> TxTrigger/1
  Divide/1 -> Data Type Conversion/1
  TxReq/1 -> Chart/1(TxReq)
  Constant/1 -> Divide/2

== system halout/HAL_OUT/CAN3/FD3_VCU5_0x155 ==
  BSCP_outputs : Inport  OutDataTypeStr=Bus: BSCP_outputs
  BOUTP_outputs : Inport  Port=2  OutDataTypeStr=Bus: BOUTP_outputs
  ActAPSPosn : Subsystem
  FrEDUSpd : Subsystem
  FrEDUSpdValid : Subsystem
  RrEDUSpd : Subsystem
  RrEDUSpdValid : Subsystem
  bus_creator : BusCreator  Inputs=5  OutDataTypeStr=Bus: DT_CAN3_SG_FD3_VCU5  NonVirtualBus=on
  bus_selector : BusSelector  OutputSignals=VOUTP_ActAPSPosn_pct
  bus_selector1 : BusSelector  OutputSignals=VOUTP_FrEDUSpd_rpm
  bus_selector2 : BusSelector  OutputSignals=VOUTP_FrEDUSpdValid_flg
  bus_selector3 : BusSelector  OutputSignals=VOUTP_RrEDUSpd_rpm
  bus_selector4 : BusSelector  OutputSignals=VOUTP_RrEDUSpdValid_flg
  FD3_VCU5 : Outport
  wires:
  BSCP_outputs/1 -> [BSCP_outputs]
  BOUTP_outputs/1 -> [BOUTP_outputs]
  [CAN3_ActAPSPosn] -> bus_creator/1  "CAN3_ActAPSPosn"
  [CAN3_Fr_EDUSpd] -> bus_creator/2  "CAN3_Fr_EDUSpd"
  [CAN3_Fr_EDUSpdValid] -> bus_creator/3  "CAN3_Fr_EDUSpdValid"
  [CAN3_Rr_EDUSpd] -> bus_creator/4  "CAN3_Rr_EDUSpd"
  [CAN3_Rr_EDUSpdValid] -> bus_creator/5  "CAN3_Rr_EDUSpdValid"
  bus_creator/1 -> FD3_VCU5/1
  ActAPSPosn/1(CAN3_ActAPSPosn) -> [CAN3_ActAPSPosn]
  FrEDUSpd/1(CAN3_Fr_EDUSpd) -> [CAN3_Fr_EDUSpd]
  FrEDUSpdValid/1(CAN3_Fr_EDUSpdValid) -> [CAN3_Fr_EDUSpdValid]
  RrEDUSpd/1(CAN3_Rr_EDUSpd) -> [CAN3_Rr_EDUSpd]
  RrEDUSpdValid/1(CAN3_Rr_EDUSpdValid) -> [CAN3_Rr_EDUSpdValid]
  bus_selector/1 -> ActAPSPosn/1(ActAPSPosn)  "<VOUTP_ActAPSPosn_pct>"
  [BOUTP_outputs] -> bus_selector/1
  bus_selector1/1 -> FrEDUSpd/1(FrEDUSpd)  "<VOUTP_FrEDUSpd_rpm>"
  [BOUTP_outputs] -> bus_selector1/1
  bus_selector2/1 -> FrEDUSpdValid/1(FrEDUSpdValid)  "<VOUTP_FrEDUSpdValid_flg>"
  [BOUTP_outputs] -> bus_selector2/1
  bus_selector3/1 -> RrEDUSpd/1(RrEDUSpd)  "<VOUTP_RrEDUSpd_rpm>"
  [BOUTP_outputs] -> bus_selector3/1
  bus_selector4/1 -> RrEDUSpdValid/1(RrEDUSpdValid)  "<VOUTP_RrEDUSpdValid_flg>"
  [BOUTP_outputs] -> bus_selector4/1

== system halout/HAL_OUT/CAN3/GW_ESC1_toNIDEC_0x152 ==
  BSCP_outputs : Inport  OutDataTypeStr=Bus: BSCP_outputs
  BOUTP_outputs : Inport  Port=2  OutDataTypeStr=Bus: BOUTP_outputs
  VehSpeedtoNidec : Subsystem
  bus_creator : BusCreator  Inputs=1  OutDataTypeStr=Bus: DT_CAN3_SG_GW_ESC1_toNIDEC  NonVirtualBus=on
  bus_selector : BusSelector  OutputSignals=VSCP_CAN3GWESC1toNIDECVehSpeedtoNidec_kph
  GW_ESC1_toNIDEC : Outport
  wires:
  BSCP_outputs/1 -> [BSCP_outputs]
  BOUTP_outputs/1 -> [BOUTP_outputs]
  [CAN3_VehSpeed_toNidec] -> bus_creator/1  "CAN3_VehSpeed_toNidec"
  bus_creator/1 -> GW_ESC1_toNIDEC/1
  VehSpeedtoNidec/1(CAN3_VehSpeed_toNidec) -> [CAN3_VehSpeed_toNidec]
  bus_selector/1 -> VehSpeedtoNidec/1(VehSpeedtoNidec)  "<VSCP_CAN3GWESC1toNIDECVehSpeedtoNidec_kph>"
  [BSCP_outputs] -> bus_selector/1

== system halout/HAL_OUT/CAN3/GW_IVI6_toNIDEC_0x49F ==
  BSCP_outputs : Inport  OutDataTypeStr=Bus: BSCP_outputs
  BOUTP_outputs : Inport  Port=2  OutDataTypeStr=Bus: BOUTP_outputs
  IVITimeDaytoNidec : Subsystem
  IVITimeHourtoNidec : Subsystem
  IVITimeMinutetoNidec : Subsystem
  IVITimeMonthtoNidec : Subsystem
  IVITimeSecondtoNidec : Subsystem
  bus_creator : BusCreator  Inputs=5  OutDataTypeStr=Bus: DT_CAN3_SG_GW_IVI6_toNIDEC  NonVirtualBus=on
  bus_selector : BusSelector  OutputSignals=VSCP_CAN3GWIVI6toNIDECIVITimeDaytoNidec_DAY
  bus_selector1 : BusSelector  OutputSignals=VSCP_CAN3GWIVI6toNIDECIVITimeHourtoNidec_hr
  bus_selector2 : BusSelector  OutputSignals=VSCP_CAN3GWIVI6toNIDECIVITimeMinutetoNidec_min
  bus_selector3 : BusSelector  OutputSignals=VSCP_CAN3GWIVI6toNIDECIVITimeMonthtoNidec_MONTH
  bus_selector4 : BusSelector  OutputSignals=VSCP_CAN3GWIVI6toNIDECIVITimeSecondtoNidec_s
  GW_IVI6_toNIDEC : Outport
  wires:
  BSCP_outputs/1 -> [BSCP_outputs]
  BOUTP_outputs/1 -> [BOUTP_outputs]
  [CAN3_IVI_Time_Day_toNidec] -> bus_creator/1  "CAN3_IVI_Time_Day_toNidec"
  [CAN3_IVI_Time_Hour_toNidec] -> bus_creator/2  "CAN3_IVI_Time_Hour_toNidec"
  [CAN3_IVI_Time_Minute_toNidec] -> bus_creator/3  "CAN3_IVI_Time_Minute_toNidec"
  [CAN3_IVI_Time_Month_toNidec] -> bus_creator/4  "CAN3_IVI_Time_Month_toNidec"
  [CAN3_IVI_Time_Second_toNidec] -> bus_creator/5  "CAN3_IVI_Time_Second_toNidec"
  bus_creator/1 -> GW_IVI6_toNIDEC/1
  IVITimeDaytoNidec/1(CAN3_IVI_Time_Day_toNidec) -> [CAN3_IVI_Time_Day_toNidec]
  IVITimeHourtoNidec/1(CAN3_IVI_Time_Hour_toNidec) -> [CAN3_IVI_Time_Hour_toNidec]
  IVITimeMinutetoNidec/1(CAN3_IVI_Time_Minute_toNidec) -> [CAN3_IVI_Time_Minute_toNidec]
  IVITimeMonthtoNidec/1(CAN3_IVI_Time_Month_toNidec) -> [CAN3_IVI_Time_Month_toNidec]
  IVITimeSecondtoNidec/1(CAN3_IVI_Time_Second_toNidec) -> [CAN3_IVI_Time_Second_toNidec]
  bus_selector/1 -> IVITimeDaytoNidec/1(IVITimeDaytoNidec)  "<VSCP_CAN3GWIVI6toNIDECIVITimeDaytoNidec_DAY>"
  [BSCP_outputs] -> bus_selector/1
  bus_selector1/1 -> IVITimeHourtoNidec/1(IVITimeHourtoNidec)  "<VSCP_CAN3GWIVI6toNIDECIVITimeHourtoNidec_hr>"
  [BSCP_outputs] -> bus_selector1/1
  bus_selector2/1 -> IVITimeMinutetoNidec/1(IVITimeMinutetoNidec)  "<VSCP_CAN3GWIVI6toNIDECIVITimeMinutetoNidec_min>"
  [BSCP_outputs] -> bus_selector2/1
  bus_selector3/1 -> IVITimeMonthtoNidec/1(IVITimeMonthtoNidec)  "<VSCP_CAN3GWIVI6toNIDECIVITimeMonthtoNidec_MONTH>"
  [BSCP_outputs] -> bus_selector3/1
  bus_selector4/1 -> IVITimeSecondtoNidec/1(IVITimeSecondtoNidec)  "<VSCP_CAN3GWIVI6toNIDECIVITimeSecondtoNidec_s>"
  [BSCP_outputs] -> bus_selector4/1
